simulink subsystem "VVI_mode"  (R2022a)
settings: Solver=VariableStepAuto  StartTime=0.0  StopTime=10.0  RelTol=1e-3
settings Model: Creator=ivanl  LastModifiedBy=tygre

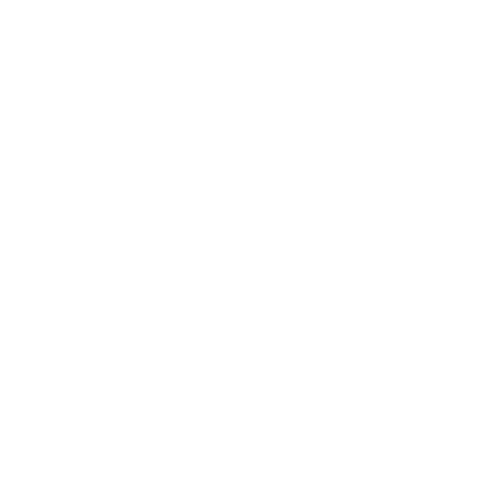
[thumbnail: Simulink's stored preview of the top-level diagram]
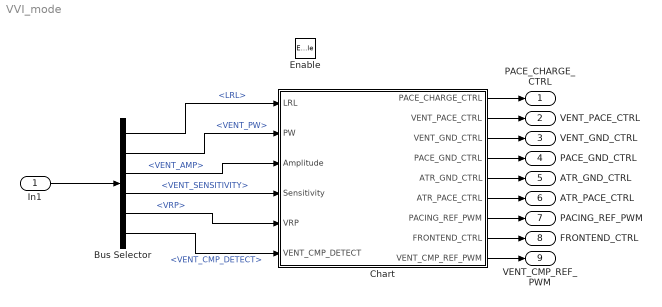
== system VVI_mode ==
  In1 : Inport
  Enable : EnablePort
  Bus Selector : BusSelector  OutputSignals=LRL,VENT_PW,VENT_AMP,VENT_SENSITIVITY,VRP,VENT_CMP_DETECT
  Chart : Stateflow chart  TreatAsAtomicUnit=on
  PACE_CHARGE_CTRL : Outport
  VENT_PACE_CTRL : Outport  Port=2
  VENT_GND_CTRL : Outport  Port=3
  PACE_GND_CTRL : Outport  Port=4
  ATR_GND_CTRL : Outport  Port=5
  ATR_PACE_CTRL : Outport  Port=6
  PACING_REF_PWM : Outport  Port=7
  FRONTEND_CTRL : Outport  Port=8
  VENT_CMP_REF_PWM : Outport  Port=9
  wires:
  In1/1 -> Bus Selector/1
  Bus Selector/1 -> Chart/1(LRL)  "<LRL>"
  Bus Selector/2 -> Chart/2(PW)  "<VENT_PW>"
  Bus Selector/3 -> Chart/3(Amplitude)  "<VENT_AMP>"
  Bus Selector/4 -> Chart/4(Sensitivity)  "<VENT_SENSITIVITY>"
  Bus Selector/5 -> Chart/5(VRP)  "<VRP>"
  Bus Selector/6 -> Chart/6(VENT_CMP_DETECT)  "<VENT_CMP_DETECT>"
  Chart/6(ATR_PACE_CTRL) -> ATR_PACE_CTRL/1
  Chart/9(VENT_CMP_REF_PWM) -> VENT_CMP_REF_PWM/1
  Chart/8(FRONTEND_CTRL) -> FRONTEND_CTRL/1
  Chart/7(PACING_REF_PWM) -> PACING_REF_PWM/1
  Chart/5(ATR_GND_CTRL) -> ATR_GND_CTRL/1
  Chart/1(PACE_CHARGE_CTRL) -> PACE_CHARGE_CTRL/1
  Chart/4(PACE_GND_CTRL) -> PACE_GND_CTRL/1
  Chart/3(VENT_GND_CTRL) -> VENT_GND_CTRL/1
  Chart/2(VENT_PACE_CTRL) -> VENT_PACE_CTRL/1

== stateflow chart VVI_mode/Chart ==
  state VVI_Charging_C22
    % Opens and closes switches as needed to charge
    % capacitor C22 (the capacitor that sends charge to the
    % heart) and discharge capacitor C21 (the capacitor
    % that sends a negative charge to the heart)
    entry:
    ATR_PACE_CTRL = false;
    VENT_PACE_CTRL = false;
    PACING_REF_PWM = Amplitude * 20;
    PACE_CHARGE_CTRL = true;
    PACE_GND_CTRL = true;
    ATR_GND_CTRL = false;
    VENT_GND_CTRL = true;
  state VVI_Pacing
    % Opens and closes switches as needed to discharge
    % capacitor C22, which paces the heart, and charge
    % capacitor C21 (the capacitor that sends to a negative
    % charge to the heart)
    entry:
    PACE_CHARGE_CTRL = false;
    PACE_GND_CTRL = true;
    ATR_PACE_CTRL = false;
    ATR_GND_CTRL = false;
    VENT_GND_CTRL = false;
    VENT_PACE_CTRL = true;
  state VVI_Sensing
    % Begins sensing for natural heart activity after waiting
    % the refractory period
    entry:
    FRONTEND_CTRL = true;
    VENT_CMP_REF_PWM = (Sensitivity)*30;
  (default) -> VVI_Charging_C22
  VVI_Pacing -> VVI_Charging_C22 : after (PW, msec)
  VVI_Sensing -> VVI_Charging_C22 [order 2] : [VENT_CMP_DETECT == true]
  VVI_Charging_C22 -> VVI_Sensing : after(VRP, msec)
  VVI_Sensing -> VVI_Pacing [order 1] : after(((60000/LRL) - VRP - PW), msec)
  data: PACE_CHARGE_CTRL output boolean; VENT_PACE_CTRL output boolean; VENT_GND_CTRL output boolean; PACE_GND_CTRL output boolean; LRL input double; PW input double; Amplitude input double; ATR_GND_CTRL output boolean; ATR_PACE_CTRL output boolean; PACING_REF_PWM output double; Sensitivity input double; VRP input double; FRONTEND_CTRL output boolean; VENT_CMP_REF_PWM output double; VENT_CMP_DETECT input boolean
